simulink model "HW5_NCEKF_sim"  (R2020a)
settings: Solver=VariableStepAuto  StartTime=0.0  StopTime=simtime  FixedStep=1  RelTol=1e-8
undefined symbols (not defined in the file): delta_t, euler_b_ECI, euler_b_LVLH, euler_LVLH_ECI, J, L_k, M_k, mag_hat_ECI, mu, P0, Q_k, quat_b_ECI, quat_b_LVLH, quat_LVLH_ECI, r, R_k, sigma_m, sigma_q, sigma_s, sun_hat_ECI, v, var_m, var_s, w_b_ECI, x_hat0
settings Model: PauseTimes=0  PacingRate=0.100000  Creator=seanthompson  LastModifiedBy=Owner
settings DebuggingCC: ArithmeticOperatorsInVariantConditions=warning
settings SFSimCC: SimUseLocalCustomCode=off  CustomCodeUndefinedFunction=UseInterfaceOnly
settings RTWCC: RTWUseLocalCustomCode=off
settings CodeAppCC: StateflowObjectComments=on

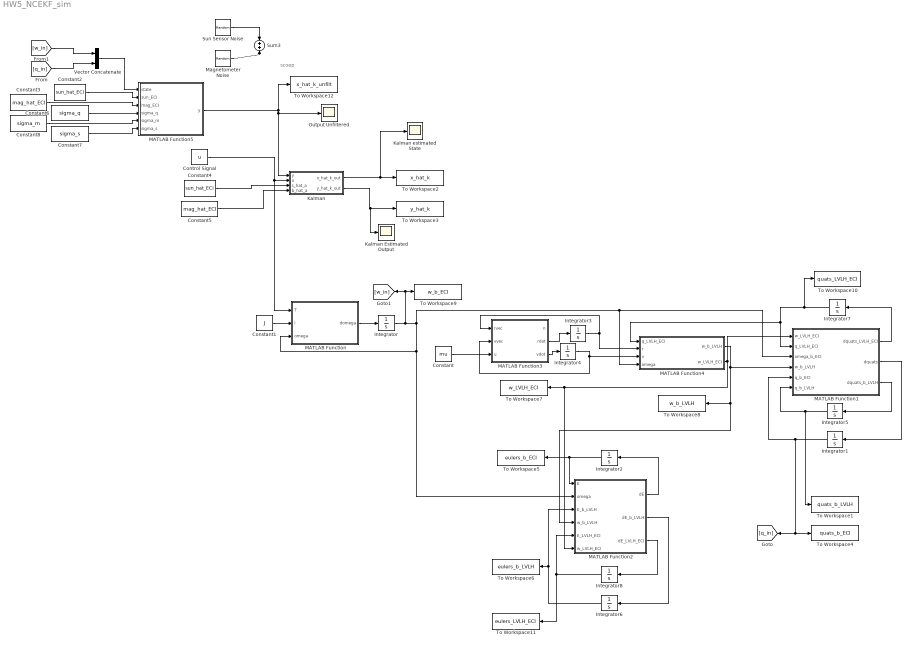
== system HW5_NCEKF_sim ==
  note: scoep
  Constant : Constant  Value=mu
  Constant1 : Constant  Value=J
  Constant2 : Constant  Value=sun_hat_ECI  VectorParams1D=off
  Constant3 : Constant  Value=mag_hat_ECI  VectorParams1D=off
  Constant4 : Constant  Value=sun_hat_ECI  VectorParams1D=off
  Constant5 : Constant  Value=mag_hat_ECI  VectorParams1D=off
  Constant6 : Constant  Value=sigma_q  VectorParams1D=off
  Constant7 : Constant  Value=sigma_s  VectorParams1D=off
  Constant8 : Constant  Value=sigma_m  VectorParams1D=off
  Control Signal : Constant  Value=u
  Integrator : Integrator  InitialCondition=w_b_ECI
  Integrator1 : Integrator  InitialCondition=quat_b_ECI
  Integrator2 : Integrator  InitialCondition=euler_b_ECI
  Integrator3 : Integrator  InitialCondition=r
  Integrator4 : Integrator  InitialCondition=v
  Integrator5 : Integrator  InitialCondition=quat_b_LVLH
  Integrator6 : Integrator  InitialCondition=euler_b_LVLH
  Integrator7 : Integrator  InitialCondition=quat_LVLH_ECI
  Integrator8 : Integrator  InitialCondition=euler_LVLH_ECI
  Kalman : Subsystem
  Kalman Estimated Output : Scope
  Kalman estimated State : Scope
  MATLAB Function : MATLAB Function  TreatAsAtomicUnit=on
  MATLAB Function1 : MATLAB Function  TreatAsAtomicUnit=on
  MATLAB Function2 : MATLAB Function  TreatAsAtomicUnit=on
  MATLAB Function3 : MATLAB Function  TreatAsAtomicUnit=on
  MATLAB Function4 : MATLAB Function  TreatAsAtomicUnit=on
  MATLAB Function5 : MATLAB Function  TreatAsAtomicUnit=on
  Magnetometer Noise : RandomNumber  Variance=var_m  SampleTime=delta_t
  Output Unfiltered : Scope
  Sum3 : Sum  Inputs=+|+
  Sun Sensor Noise : RandomNumber  Variance=var_s  SampleTime=delta_t
  To Workspace1 : ToWorkspace  VariableName=quats_b_LVLH  SaveFormat=Timeseries  SampleTime=-1
  To Workspace10 : ToWorkspace  VariableName=quats_LVLH_ECI  SaveFormat=Timeseries  SampleTime=-1
  To Workspace11 : ToWorkspace  VariableName=eulers_LVLH_ECI  SaveFormat=Timeseries  SampleTime=-1
  To Workspace12 : ToWorkspace  VariableName=x_hat_k_unfilt  SaveFormat=Timeseries  SampleTime=-1
  To Workspace2 : ToWorkspace  VariableName=x_hat_k  SaveFormat=Timeseries  SampleTime=-1
  To Workspace3 : ToWorkspace  VariableName=y_hat_k  SaveFormat=Timeseries  SampleTime=-1
  To Workspace4 : ToWorkspace  VariableName=quats_b_ECI  SaveFormat=Timeseries  SampleTime=-1
  To Workspace5 : ToWorkspace  VariableName=eulers_b_ECI  SaveFormat=Timeseries  SampleTime=-1
  To Workspace6 : ToWorkspace  VariableName=eulers_b_LVLH  SaveFormat=Timeseries  SampleTime=-1
  To Workspace7 : ToWorkspace  VariableName=w_LVLH_ECI  SaveFormat=Timeseries  SampleTime=-1
  To Workspace8 : ToWorkspace  VariableName=w_b_LVLH  SaveFormat=Timeseries  SampleTime=-1
  To Workspace9 : ToWorkspace  VariableName=w_b_ECI  SaveFormat=Timeseries  SampleTime=-1
  Vector Concatenate : Concatenate  Mode=Multidimensional array
  wires:
  MATLAB Function5/1(y) -> Kalman/1(y), Output Unfiltered/1, To Workspace12/1
  Kalman/1(x_hat_k_out) -> Kalman estimated State/1, To Workspace2/1
  Sun Sensor Noise/1 -> Sum3/1
  Magnetometer Noise/1 -> Sum3/2
  Control Signal/1 -> MATLAB Function/1(T), Kalman/2(u)
  MATLAB Function2/3(dE_LVLH_ECI) -> Integrator8/1
  Integrator6/1 -> To Workspace6/1, MATLAB Function2/3(E_b_LVLH)
  Integrator7/1 -> To Workspace10/1, MATLAB Function4/1(q_LVLH_ECI), MATLAB Function1/2(q_LVLH_ECI)
  MATLAB Function3/2(rdot) -> Integrator3/1
  Integrator/1 -> [w_in], To Workspace9/1, MATLAB Function/3(omega), MATLAB Function2/2(omega), MATLAB Function4/4(omega), MATLAB Function1/3(omega_b_ECI)
  MATLAB Function/1(domega) -> Integrator/1
  Integrator2/1 -> To Workspace5/1, MATLAB Function2/1(E)
  Constant1/1 -> MATLAB Function/2(I)
  MATLAB Function2/2(dE_b_LVLH) -> Integrator6/1
  MATLAB Function4/2(w_LVLH_ECI) -> MATLAB Function1/1(w_LVLH_ECI), MATLAB Function2/6(w_LVLH_ECI), To Workspace7/1
  MATLAB Function4/1(w_b_LVLH) -> MATLAB Function2/4(w_b_LVLH), To Workspace8/1, MATLAB Function1/4(w_b_LVLH)
  MATLAB Function2/1(dE) -> Integrator2/1
  Constant/1 -> MATLAB Function3/3(u)
  MATLAB Function1/1(dquats_LVLH_ECI) -> Integrator7/1
  Integrator4/1 -> MATLAB Function4/3(v), MATLAB Function3/2(vvec)
  MATLAB Function1/3(dquats_b_LVLH) -> Integrator5/1
  Integrator3/1 -> MATLAB Function3/1(rvec), MATLAB Function4/2(r)
  Integrator8/1 -> To Workspace11/1, MATLAB Function2/5(E_LVLH_ECI)
  MATLAB Function3/3(vdot) -> Integrator4/1
  MATLAB Function1/2(dquats) -> Integrator1/1
  Integrator5/1 -> MATLAB Function1/6(q_b_LVLH), To Workspace1/1
  Constant2/1 -> MATLAB Function5/2(sun_ECI)
  Constant3/1 -> MATLAB Function5/3(mag_ECI)
  Integrator1/1 -> MATLAB Function1/5(q_b_ECI), [q_in], To Workspace4/1
  Vector Concatenate/1 -> MATLAB Function5/1(state)
  [q_in] -> Vector Concatenate/2
  [w_in] -> Vector Concatenate/1
  Constant5/1 -> Kalman/4(b_hat_a)
  Constant4/1 -> Kalman/3(s_hat_a)
  Constant6/1 -> MATLAB Function5/4(sigma_q)
  Constant8/1 -> MATLAB Function5/5(sigma_m)
  Constant7/1 -> MATLAB Function5/6(sigma_s)
  Kalman/2(y_hat_k_out) -> Kalman Estimated Output/1, To Workspace3/1

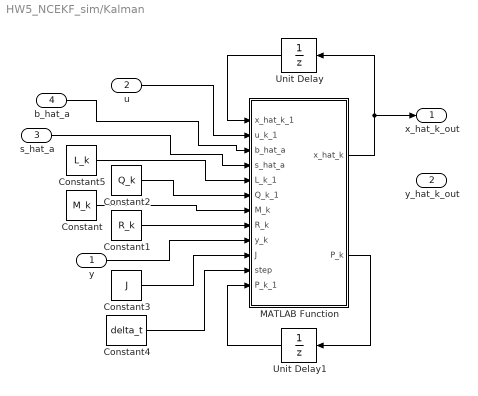
== system HW5_NCEKF_sim/Kalman ==
  y : Inport
  u : Inport  Port=2
  s_hat_a : Inport  Port=3
  b_hat_a : Inport  Port=4
  Constant : Constant  Value=M_k  VectorParams1D=off
  Constant1 : Constant  Value=R_k  VectorParams1D=off
  Constant2 : Constant  Value=Q_k  VectorParams1D=off
  Constant3 : Constant  Value=J  VectorParams1D=off
  Constant4 : Constant  Value=delta_t
  Constant5 : Constant  Value=L_k  VectorParams1D=off
  MATLAB Function : MATLAB Function  TreatAsAtomicUnit=on
  Unit Delay : UnitDelay  InitialCondition=x_hat0  SampleTime=delta_t  HasFrameUpgradeWarning=on
  Unit Delay1 : UnitDelay  InitialCondition=P0  SampleTime=delta_t  HasFrameUpgradeWarning=on
  x_hat_k_out : Outport
  y_hat_k_out : Outport  Port=2
  wires:
  MATLAB Function/1(x_hat_k) -> Unit Delay/1, x_hat_k_out/1
  MATLAB Function/2(P_k) -> Unit Delay1/1
  Unit Delay1/1 -> MATLAB Function/12(P_k_1)
  u/1 -> MATLAB Function/2(u_k_1)
  Unit Delay/1 -> MATLAB Function/1(x_hat_k_1)
  y/1 -> MATLAB Function/9(y_k)
  Constant2/1 -> MATLAB Function/6(Q_k_1)
  Constant/1 -> MATLAB Function/7(M_k)
  Constant1/1 -> MATLAB Function/8(R_k)
  Constant3/1 -> MATLAB Function/10(J)
  Constant4/1 -> MATLAB Function/11(step)
  Constant5/1 -> MATLAB Function/5(L_k_1)
  s_hat_a/1 -> MATLAB Function/4(s_hat_a)
  b_hat_a/1 -> MATLAB Function/3(b_hat_a)

== matlab function HW5_NCEKF_sim/MATLAB Function4 ==
  data: q_LVLH_ECI input; r input; w_b_LVLH output; v input; omega input; w_LVLH_ECI output
function [w_b_LVLH,w_LVLH_ECI] = omega_b_LVLH(q_LVLH_ECI,r,v,omega)
C_LVLH_ECI = Functions.quat2rot(q_LVLH_ECI);
w_LVLH_ECI = C_LVLH_ECI*(cross(r,v)/norm(r)^2); % apply ECI to LVLH transformation matrix
w_b_LVLH = omega - w_LVLH_ECI;

% possibly needs rotation matrix

== matlab function HW5_NCEKF_sim/MATLAB Function ==
  data: T input; I input; domega output; omega input
function domega = DYNAMICS(T,I,omega)
    
domega = I\(T-Functions.vec2cross(omega)*I*omega);
% domega = I\(T-cross(omega,I*omega));

end

== matlab function HW5_NCEKF_sim/Kalman/MATLAB Function ==
  data: x_hat_k_1 input; u_k_1 input; b_hat_a input; s_hat_a input; L_k_1 input; Q_k_1 input; M_k input; R_k input; y_k input; J input; x_hat_k output; step input; P_k_1 input; P_k output
function [x_hat_k,  P_k] = K(x_hat_k_1,u_k_1,b_hat_a,s_hat_a,L_k_1,Q_k_1,M_k,R_k,y_k,J,step,P_k_1)
% Norm-Constrained Extended Kalman Filter
% Based on DeReuter's Spacecraft ADC Example 25.3

% Extract angular velocity and quaternion from state
omega_hat_k_1 = x_hat_k_1(1:3);
q_hat_k_1 = x_hat_k_1(4:7);

% Extract quaternion components
eta = q_hat_k_1(4);
eps = q_hat_k_1(1:3);

%% Predictor

% Set Kalman constants at this step
F_k_1 = eye(7) + step*[pinv(J)*(-Functions.vec2cross(omega_hat_k_1)*J+Functions.vec2cross(J*omega_hat_k_1)) zeros(3)                               zeros([3 1]);
                       0.5*(eta*eye(3)+Functions.vec2cross(eps))                                          -0.5*Functions.vec2cross(omega_hat_k_1) 0.5*omega_hat_k_1;
                      -0.5*eps'                                                                           -0.5*omega_hat_k_1'                     0];
x_hat_k_minus = f(x_hat_k_1,u_k_1,step,J); % f_k_1 is some function of x_hat_k_1, u_k_1, and 0

P_k_minus = F_k_1*P_k_1*F_k_1' + L_k_1*Q_k_1*L_k_1';

% Extract Pk sub-matrices
P_k_minus_1 = P_k_minus(:,1:3);
P_k_minus_2 = P_k_minus(:,4:7);
P_k_ww_minus = P_k_minus(1:3,1:3);
P_k_wq_minus = P_k_minus(1:3,4:7);
P_k_qw_minus = P_k_minus(4:7,1:3);
P_k_qq_minus = P_k_minus(4:7,4:7);

%% Corrector
w_hat_k_minus = x_hat_k_minus(1:3);
q_hat_k_minus = x_hat_k_minus(4:7);

% more constants

% Big H constant, uses Y-bar of previous state
H_k = [zeros(3) Y_bar(b_hat_a,q_hat_k_1); % for magnetic field and sun
       zeros(3) Y_bar(s_hat_a,q_hat_k_1)];
W_k = H_k*P_k_minus*H_k' + M_k*R_k*M_k';
K_w_k = P_k_minus_1'*H_k'*pinv(W_k); 

% Little h constant, uses Y of estimated state
h_k = [zeros(3) Y(b_hat_a,q_hat_k_minus);
       zeros(3) Y(s_hat_a,q_hat_k_minus)]*x_hat_k_minus;

% Calculate new estimated angular velocity
r_k = y_k - h_k;
r_italic_k = r_k'*pinv(W_k)*r_k;
omega_hat_k = w_hat_k_minus + K_w_k*r_k; % Updated angular velocity

% Calculate new estimated quaternion
K_q_tilde_k = P_k_minus_2'*H_k'*pinv(W_k);
q_tilde_k = q_hat_k_minus + K_q_tilde_k*r_k;
K_q_k = K_q_tilde_k + 1/r_italic_k*(1/norm(q_tilde_k)-1)*q_tilde_k*r_k'*pinv(W_k);
q_hat_k = q_hat_k_minus + K_q_k*r_k; % Updated quaternion

Pww = P_k_ww_minus - K_w_k*H_k*P_k_minus_1 - P_k_minus_1'*H_k'*K_w_k' + K_w_k*W_k*K_w_k';
Pwq = P_k_wq_minus - K_w_k*H_k*P_k_minus_2 - P_k_minus_1'*H_k'*K_q_k' + K_w_k*W_k*K_q_k';
Pqw = P_k_qw_minus - K_q_k*H_k*P_k_minus_1 - P_k_minus_2'*H_k'*K_w_k' + K_q_k*W_k*K_w_k';
Pqq = P_k_qq_minus - K_q_k*H_k*P_k_minus_2 - P_k_minus_2'*H_k'*K_q_k' + K_q_k*W_k*K_q_k';

P_k = [Pww Pwq
       Pqw Pqq];
x_hat_k = [omega_hat_k; q_hat_k];

end

%%%%%%%%%%%%%%%%%%%%%%%%
% SUPPORTING FUNCTIONS %
%%%%%%%%%%%%%%%%%%%%%%%%

function x_k = f(x_k_1,u_k_1,T,J)
omega_k_1 = x_k_1(1:3);
quat_k_1 = x_k_1(4:7);

eps = quat_k_1(1:3);
eta = quat_k_1(4);

x_k = x_k_1 + T*[pinv(J)*(-Functions.vec2cross(omega_k_1)*J*omega_k_1 + u_k_1);
                 0.5*(eta*eye(3)+Functions.vec2cross(eps))*omega_k_1;
                -0.5*eps'*omega_k_1];
end

function Y_out = Y(a,q)
% Essentially a rotation of a via q
eta = q(4);
eps = q(1:3);
Y_out = [eta*eye(3)-Functions.vec2cross(eps) -eps]*[Functions.vec2cross(a) a; -a' 0];   
end

function Y_bar_out = Y_bar(a,q)
% Same as Y_out but with an additional step for 'true'
eta = q(4);
eps = q(1:3);
Y_b = [eta*eye(3)-Functions.vec2cross(eps) -eps]*[Functions.vec2cross(a) a;-a' 0];
Y_bar_out = Y_b + [Functions.vec2cross(Functions.vec2cross(a)*eps+a*eta)+a'*eps*eye(3) (Functions.vec2cross(a)*eps+a*eta)];
end

== matlab function HW5_NCEKF_sim/MATLAB Function1 ==
  data: w_LVLH_ECI input; q_LVLH_ECI input; dquats_LVLH_ECI output; omega_b_ECI input; dquats output; w_b_LVLH input; q_b_ECI input; q_b_LVLH input; dquats_b_LVLH output
function [dquats_LVLH_ECI,dquats,dquats_b_LVLH] = quats(w_LVLH_ECI,q_LVLH_ECI,omega_b_ECI,w_b_LVLH,q_b_ECI,q_b_LVLH)

% ECI to Body
eps = q_b_ECI(1:3,1);
eta = q_b_ECI(4,1);

epsilonDot = 0.5*(eta*eye(3)+Functions.vec2cross(eps))*omega_b_ECI;
etaDot = -0.5*eps'*omega_b_ECI;

% LVLH to Body
eps_b_LVLH = q_b_LVLH(1:3);
eta_b_LVLH = q_b_LVLH(4);
epsilonDot_b_LVLH = 0.5*(eta_b_LVLH*eye(3)+Functions.vec2cross(eps_b_LVLH))*w_b_LVLH;
etaDot_b_LVLH = -0.5*eps_b_LVLH'*w_b_LVLH;

% ECI to LVLH
eps_LVLH_ECI = q_LVLH_ECI(1:3);
eta_LVLH_ECI = q_LVLH_ECI(4);
epsilonDot_LVLH_ECI = 0.5*(eta_LVLH_ECI*eye(3)+Functions.vec2cross(eps_LVLH_ECI))*w_LVLH_ECI;
etaDot_LVLH_ECI = -0.5*eps_LVLH_ECI'*w_LVLH_ECI;

dquats = [epsilonDot; etaDot];
dquats_b_LVLH = [epsilonDot_b_LVLH; etaDot_b_LVLH];
dquats_LVLH_ECI = [epsilonDot_LVLH_ECI; etaDot_LVLH_ECI];

== matlab function HW5_NCEKF_sim/MATLAB Function2 ==
  data: E input; omega input; dE output; E_b_LVLH input; w_b_LVLH input; dE_b_LVLH output; E_LVLH_ECI input; w_LVLH_ECI input; dE_LVLH_ECI output
function [dE,dE_b_LVLH,dE_LVLH_ECI]  = euler(E,omega,E_b_LVLH,w_b_LVLH,E_LVLH_ECI,w_LVLH_ECI)

% ECI to Body
place = 1/cos(E(2))* [cos(E(2)) sin(E(1))*sin(E(2)) cos(E(1))*sin(E(2)); 
                        0          cos(E(1))*cos(E(2)) -sin(E(1))*cos(E(2)); 
                        0          sin(E(1))                  cos(E(1))];

dE =place*omega;

% LVLH to Body
place_b_LVLH = 1/cos(E_b_LVLH(2))* [cos(E_b_LVLH(2)) sin(E_b_LVLH(1))*sin(E_b_LVLH(2)) cos(E_b_LVLH(1))*sin(E_b_LVLH(2)); 
                        0          cos(E_b_LVLH(1))*cos(E_b_LVLH(2)) -sin(E_b_LVLH(1))*cos(E_b_LVLH(2)); 
                        0          sin(E_b_LVLH(1))                  cos(E_b_LVLH(1))];

dE_b_LVLH =place_b_LVLH*w_b_LVLH;

% ECI to LVLH
place_LVLH_ECI = 1/cos(E_LVLH_ECI(2))* [cos(E_LVLH_ECI(2)) sin(E_LVLH_ECI(1))*sin(E_LVLH_ECI(2)) cos(E_LVLH_ECI(1))*sin(E_LVLH_ECI(2)); 
                        0          cos(E_LVLH_ECI(1))*cos(E_LVLH_ECI(2)) -sin(E_LVLH_ECI(1))*cos(E_LVLH_ECI(2)); 
                        0          sin(E_LVLH_ECI(1))                  cos(E_LVLH_ECI(1))];

dE_LVLH_ECI =place_LVLH_ECI*w_LVLH_ECI;

== matlab function HW5_NCEKF_sim/MATLAB Function3 ==
  data: n output; rvec input; rdot output; vvec input; u input; vdot output
function [n,rdot,vdot] = rvProp(rvec,vvec,u)

rmag = norm(rvec);

% Find angular momentum
hvec = cross(rvec,vvec);
hmag = norm(hvec);

% Find eccentricity
eccvec = 1/u*(cross(vvec,hvec) - u*(rvec/rmag));
eccmag = norm(eccvec);

% Find semimajor axis
if eccmag < 1 && eccmag > 0
    a = (hmag^2/u)*(1/(1-eccmag^2));
elseif eccmag == 0
    a = rmag*2;
else
    a = -(hmag^2/u)*(1/(eccmag^2-1));
end

% Calculate period in seconds and mean motion in rad/s
T = 2*pi/sqrt(u)*(a)^(3/2); 
n = 2*pi/T;

rdot = vvec;
vdot = -u*rvec/(norm(rvec)^3);

end

== matlab function HW5_NCEKF_sim/MATLAB Function5 ==
  data: state input; y output; sun_ECI input; mag_ECI input; sigma_q input; sigma_m input; sigma_s input
function y = Yq(state,sun_ECI,mag_ECI,sigma_q,sigma_m,sigma_s)
% Calculate Y(a,q) matrix times the state WITHOUT process noise

q = state(4:7);
eps = q(1:3);
eta = q(4);

% Calculate Y(a,q) for magnetometer and sun sensor
Y_b = [eta*eye(3)-Functions.vec2cross(eps) -eps]*[Functions.vec2cross(mag_ECI) mag_ECI;
                                                      -mag_ECI'                    0];
Y_s = [eta*eye(3)-Functions.vec2cross(eps) -eps]*[Functions.vec2cross(sun_ECI) sun_ECI;
                                                      -sun_ECI'                    0];

coder.extrinsic('randn');
v_k = zeros([6 1]); %#ok<*PREALL> simulink needs this to determine variable size
v_k = randn(6,1)*sigma_q;   
m_k = zeros([6 1]);
m_k = [randn(3,1)*sigma_m;
       randn(3,1)*sigma_s];
y = [zeros(3) Y_b
     zeros(3) Y_s]*state + m_k + v_k; % measurement with measurement and process noise
end
